simulink model "simulator_AMICAS_M2022a"  (R2024a)
settings: Solver=ode3  StartTime=0.0  StopTime=Tsim  FixedStep=ST  RelTol=1e-3
values from neighbouring files (symbols this model uses):
  alpha_G = 15.03    [anesthesia_model_AMICAS.m]
  alpha_RG = 0.33    [anesthesia_model_AMICAS.m]
  beta_M = 10.74    [anesthesia_model_AMICAS.m]
  C50N = 3.2425    [anesthesia_model_AMICAS.m]
  C50P_G = 7.66    [anesthesia_model_AMICAS.m]
  C50P_M = 7.53    [anesthesia_model_AMICAS.m]
  C50P_RG = 8.26    [anesthesia_model_AMICAS.m]
  C50Pco = 8    [hemodyn_model_AMICAS.m]
  C50Pmap = 6    [hemodyn_model_AMICAS.m]
  C50R_G = 149.62    [anesthesia_model_AMICAS.m]
  C50R_M = 160.25    [anesthesia_model_AMICAS.m]
  C50Rco = 12    [hemodyn_model_AMICAS.m]
  C50Rmap = 17    [hemodyn_model_AMICAS.m]
  Cobasis = 5    [hemodyn_model_AMICAS.m]
  E0_G = 93.97    [anesthesia_model_AMICAS.m]
  E0_M = 93.97    [anesthesia_model_AMICAS.m]
  E0_RG = 93.97    [anesthesia_model_AMICAS.m]
  Emax_G = E0_G    (= 93.97)    [anesthesia_model_AMICAS.m]
  Emax_M = E0_M    (= 93.97)    [anesthesia_model_AMICAS.m]
  Emax_RG = E0_RG    (= 93.97)    [anesthesia_model_AMICAS.m]
  EmaxPco = 5    [hemodyn_model_AMICAS.m]
  EmaxPmap = 5    [hemodyn_model_AMICAS.m]
  EmaxRco = 5    [hemodyn_model_AMICAS.m]
  EmaxRmap = 70    [hemodyn_model_AMICAS.m]
  gainPco = 10    [hemodyn_model_AMICAS.m]
  gainPmap = 15    [hemodyn_model_AMICAS.m]
  gainRco = 10    [hemodyn_model_AMICAS.m]
  gainRmap = 10    [hemodyn_model_AMICAS.m]
  gamma_G = 4.07    [anesthesia_model_AMICAS.m]
  gamma_M = 4.13    [anesthesia_model_AMICAS.m]
  gamma_RG = 3.59    [anesthesia_model_AMICAS.m]
  gammaN = 2.6677    [anesthesia_model_AMICAS.m]
  gammaPco = 4.5    [hemodyn_model_AMICAS.m]
  gammaPmap = 4.5    [hemodyn_model_AMICAS.m]
  gammaRco = 4.5    [hemodyn_model_AMICAS.m]
  gammaRmap = 4.5    [hemodyn_model_AMICAS.m]
  k0Pco = 0.81    [hemodyn_model_AMICAS.m]
  k0Pmap = 0.81    [hemodyn_model_AMICAS.m]
  k0Rco = 0.51    [hemodyn_model_AMICAS.m]
  k0Rmap = 0.31    [hemodyn_model_AMICAS.m]
  k1Pco = 0.81    [hemodyn_model_AMICAS.m]
  k1Pmap = 0.61    [hemodyn_model_AMICAS.m]
  k1Rco = 0.51    [hemodyn_model_AMICAS.m]
  k1Rmap = 0.31    [hemodyn_model_AMICAS.m]
  MAPbasis = 80    [hemodyn_model_AMICAS.m]
undefined symbols (not defined in the file or in its folder): Anest_loop, Dist_type, patient, RSM_type, Ts
libraries: cstblocks x12
settings Model: Creator=Merigo  LastModifiedBy=jarverha
settings SolverCC: AlgebraicLoopSolver=TrustRegion
settings DataIOCC: LimitDataPoints=on  SaveFormat=Array  SignalLoggingSaveFormat=ModelDataLogs  ReturnWorkspaceOutputs=off
settings OptimizationCC: BlockReduction=off  BooleanDataType=off  ReuseModelBlockBuffer=off  ExpressionDepthLimit=2147483647  LifeSpan=inf
settings DebuggingCC: SaveWithParameterizedLinksMsg=none  UnderspecifiedInitializationDetection=Classic  MergeDetectMultiDrivingBlocksExec=none  SignalResolutionControl=TryResolveAllWithWarning  MultiTaskDSMMsg=warning  MultiTaskCondExecSysMsg=none  UnconnectedInputMsg=warning  UnconnectedOutputMsg=warning  UnconnectedLineMsg=warning  StateNameClashWarn=warning  SFUnexpectedBacktrackingDiag=warning  SFNoUnconditionalDefaultTransitionDiag=warning  SFExecutionAtInitializationDiag=none  ArithmeticOperatorsInVariantConditions=warning
settings HardwareCC: ProdBitPerPointer=32  ProdBitPerSizeT=32  ProdBitPerPtrDiffT=32  ProdLargestAtomicFloat=None  ProdIntDivRoundTo=Undefined  ProdEndianess=Unspecified  ProdWordSize=32  ProdHWDeviceType=32-bit Generic  TargetUnknown=on
settings ModelReferenceCC: EnableRefExpFcnMdlSchedulingChecks=on  PropagateSignalLabelsOutOfModel=off
settings SFSimCC: SimUseLocalCustomCode=off  CustomCodeUndefinedFunction=UseInterfaceOnly
settings RTWCC: RTWUseLocalCustomCode=off  GPUComputeCapability=3.5  DLArmComputeVersion=19.05
settings CodeAppCC: StateflowObjectComments=on
settings GRTTargetCC: TargetLangStandard=C89/C90 (ANSI)
settings ConfigComp: CovMetricSettings=dw  CovSaveCumulativeToWorkspaceVar=on  CovSaveSingleToWorkspaceVar=on  CovExternalEMLEnable=off

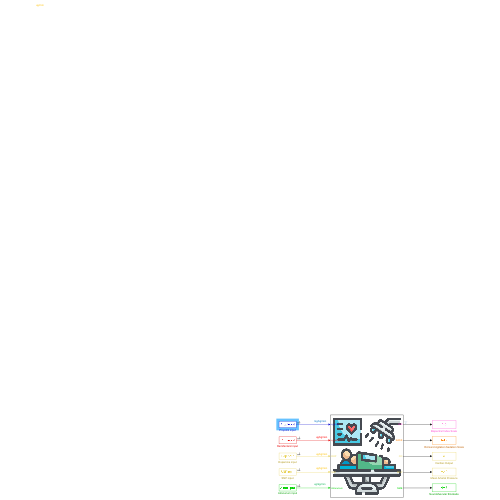
[thumbnail: Simulink's stored preview of the top-level diagram]
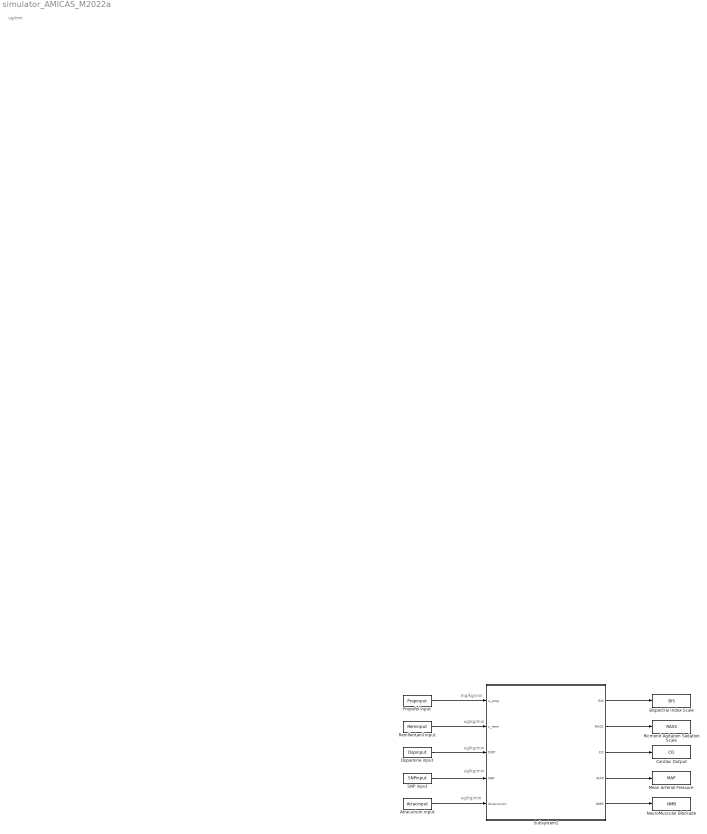
== system simulator_AMICAS_M2022a ==
  note: ug/kg/min
  note: mg/kg/min
  note: ug/min
  note: ug/kg/min
  note: ug/kg/min
  note: ug/kg/min
  Atracurium input : FromWorkspace  VariableName=Atracinput  Interpolate=off  OutputAfterFinalValue=Setting to zero
  Bispectral Index Scale : ToWorkspace  VariableName=BIS  SaveFormat=Timeseries  SampleTime=-1
  Cardiac Output : ToWorkspace  VariableName=CO  SaveFormat=Timeseries  SampleTime=-1
  Dopamine input : FromWorkspace  VariableName=Dopinput  Interpolate=off  OutputAfterFinalValue=Setting to zero
  Mean Arterial Pressure : ToWorkspace  VariableName=MAP  SaveFormat=Timeseries  SampleTime=-1
  NeuroMuscular Blockade : ToWorkspace  VariableName=NMB  SaveFormat=Timeseries  SampleTime=-1
  Propofol input : FromWorkspace  VariableName=Propinput  Interpolate=off  OutputAfterFinalValue=Setting to zero
  Remifentanil input : FromWorkspace  VariableName=Reminput  Interpolate=off  OutputAfterFinalValue=Setting to zero
  Ricmond Agitation Sedation Scale : ToWorkspace  VariableName=RASS  SaveFormat=Timeseries  SampleTime=-1
  SNP input : FromWorkspace  VariableName=SNPinput  Interpolate=off  OutputAfterFinalValue=Setting to zero
  Subsystem2 : Subsystem
      mask Display: image('$imagefile');
  wires:
  Propofol input/1 -> Subsystem2/1(u_prop)
  Subsystem2/2(RASS) -> Ricmond Agitation Sedation Scale/1
  Subsystem2/3(CO) -> Cardiac Output/1
  Subsystem2/4(MAP) -> Mean Arterial Pressure/1
  Subsystem2/5(NMB) -> NeuroMuscular Blockade/1
  Atracurium input/1 -> Subsystem2/5(Atracurium)
  Subsystem2/1(BIS) -> Bispectral Index Scale/1
  Remifentanil input/1 -> Subsystem2/2(u_remi)
  Dopamine input/1 -> Subsystem2/3(DOP)
  SNP input/1 -> Subsystem2/4(SNP)

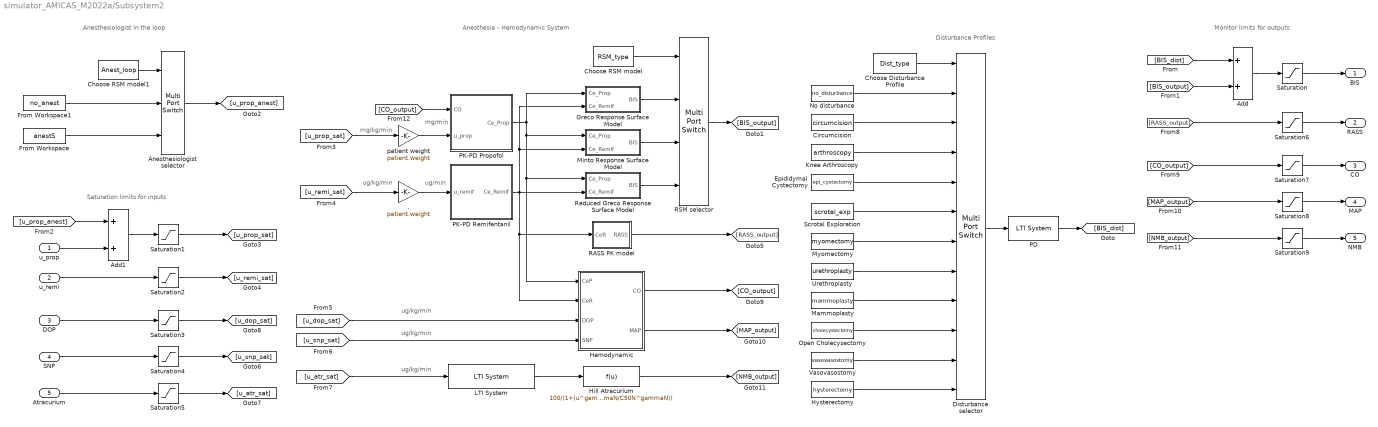
== system simulator_AMICAS_M2022a/Subsystem2 ==
  note: Disturbance Profiles
  note: Anesthesia - Hemodynamic System
  note: ug/kg/min
  note: ug/kg/min
  note: ug/kg/min
  note: ug/kg/min
  note: mg/kg/min
  note: Anesthesiologist in the loop
  note: ug/min
  note: mg/min
  note: Saturation limits for inputs
  note: Monitor limits for outputs
  u_prop : Inport
  u_remi : Inport  Port=2
  DOP : Inport  Port=3
  SNP : Inport  Port=4
  Atracurium : Inport  Port=5
  . : Gain  Gain=patient.weight
  Add : Sum
  Add1 : Sum
  Anesthesiologist selector : MultiPortSwitch  DataPortOrder=Specify indices  Inputs=2  DataPortIndices={1,2}  SaturateOnIntegerOverflow=off  InputSameDT=off
  Choose Disturbance Profile : Constant  Value=Dist_type
  Choose RSM model : Constant  Value=RSM_type
  Choose RSM model1 : Constant  Value=Anest_loop
  Circumcision : FromWorkspace  VariableName=circumcision  Interpolate=off  OutputAfterFinalValue=Setting to zero
  Disturbance selector : MultiPortSwitch  DataPortOrder=Specify indices  Inputs=10  DataPortIndices={1,2,3,4,5,6,7,8,9,10,11}  SaturateOnIntegerOverflow=off  InputSameDT=off
  Epididymal Cystectomy : FromWorkspace  VariableName=epi_cystectomy  Interpolate=off  OutputAfterFinalValue=Setting to zero
  From Workspace : FromWorkspace  VariableName=anestS
  From Workspace1 : FromWorkspace  VariableName=no_anest
  Greco Response Surface Model : Subsystem
  Hemodynamic : Subsystem
  Hill Atracurium : Fcn  Expr=100/(1+(u^gammaN/C50N^gammaN))
  Hysterectomy : FromWorkspace  VariableName=hysterectomy  Interpolate=off  OutputAfterFinalValue=Setting to zero
  Knee Arthroscopy : FromWorkspace  VariableName=arthroscopy  Interpolate=off  OutputAfterFinalValue=Setting to zero
  LTI System : cstblocks/LTI System  sys=sysNMB  IC=[]  PadeOrder=0
  Mammoplasty : FromWorkspace  VariableName=mammoplasty  Interpolate=off  OutputAfterFinalValue=Setting to zero
  Minto Response Surface Model : Subsystem
  Myomectomy : FromWorkspace  VariableName=myomectomy  Interpolate=off  OutputAfterFinalValue=Setting to zero
  No disturbance : FromWorkspace  VariableName=no_disturbance  Interpolate=off  OutputAfterFinalValue=Setting to zero
  Open Cholecysectomy : FromWorkspace  VariableName=cholecystectomy  Interpolate=off  OutputAfterFinalValue=Setting to zero
  PD : cstblocks/LTI System  sys=CPmodelP  IC=[]  PadeOrder=0
  PK-PD Propofol : Subsystem
  PK-PD Remifentanil : Subsystem
  RASS PK model : Subsystem
  RSM selector : MultiPortSwitch  DataPortOrder=Specify indices  SaturateOnIntegerOverflow=off  InputSameDT=off
  Reduced Greco Response Surface Model : Subsystem
  Saturation : Saturate  UpperLimit=100  LowerLimit=0
  Saturation1 : Saturate  UpperLimit=2.5  LowerLimit=0
  Saturation2 : Saturate  UpperLimit=4  LowerLimit=0
  Saturation3 : Saturate  UpperLimit=20  LowerLimit=0
  Saturation4 : Saturate  UpperLimit=10  LowerLimit=0
  Saturation5 : Saturate  UpperLimit=29.5  LowerLimit=0
  Saturation6 : Saturate  UpperLimit=4  LowerLimit=-5
  Saturation7 : Saturate  UpperLimit=40  LowerLimit=0
  Saturation8 : Saturate  UpperLimit=150  LowerLimit=0
  Saturation9 : Saturate  UpperLimit=100  LowerLimit=0
  Scrotal Exploration : FromWorkspace  VariableName=scrotal_exp  Interpolate=off  OutputAfterFinalValue=Setting to zero
  Urethroplasty : FromWorkspace  VariableName=urethroplasty  Interpolate=off  OutputAfterFinalValue=Setting to zero
  Vasovasostomy : FromWorkspace  VariableName=vasovasostomy  Interpolate=off  OutputAfterFinalValue=Setting to zero
  patient weight : Gain  Gain=patient.weight
  BIS : Outport
  RASS : Outport  Port=2
  CO : Outport  Port=3
  MAP : Outport  Port=4
  NMB : Outport  Port=5
  wires:
  PK-PD Remifentanil/1(Ce_Remif) -> Minto Response Surface Model/2(Ce_Remif), Greco Response Surface Model/2(Ce_Remif), Hemodynamic/2(CeR), RASS PK model/1(CeR), Reduced Greco Response Surface Model/2(Ce_Remif)
  PK-PD Propofol/1(Ce_Prop) -> Hemodynamic/1(CeP), Reduced Greco Response Surface Model/1(Ce_Prop), Minto Response Surface Model/1(Ce_Prop), Greco Response Surface Model/1(Ce_Prop)
  RASS PK model/1(RASS) -> [RASS_output]
  Hill Atracurium/1 -> [NMB_output]
  [u_atr_sat] -> LTI System/1
  LTI System/1 -> Hill Atracurium/1
  [u_dop_sat] -> Hemodynamic/3(DOP)
  [u_snp_sat] -> Hemodynamic/4(SNP)
  Hemodynamic/1(CO) -> [CO_output]
  Hemodynamic/2(MAP) -> [MAP_output]
  From Workspace/1 -> Anesthesiologist selector/3
  [u_remi_sat] -> ./1
  Reduced Greco Response Surface Model/1(BIS) -> RSM selector/4
  Greco Response Surface Model/1(BIS) -> RSM selector/2
  Minto Response Surface Model/1(BIS) -> RSM selector/3
  RSM selector/1 -> [BIS_output]
  Choose RSM model/1 -> RSM selector/1
  Add/1 -> Saturation/1
  Disturbance selector/1 -> PD/1
  No disturbance/1 -> Disturbance selector/2
  [BIS_dist] -> Add/1
  Circumcision/1 -> Disturbance selector/3
  Choose Disturbance Profile/1 -> Disturbance selector/1
  PD/1 -> [BIS_dist]
  [BIS_output] -> Add/2
  Choose RSM model1/1 -> Anesthesiologist selector/1
  Anesthesiologist selector/1 -> [u_prop_anest]
  Myomectomy/1 -> Disturbance selector/7
  Urethroplasty/1 -> Disturbance selector/8
  Mammoplasty/1 -> Disturbance selector/9
  Open Cholecysectomy/1 -> Disturbance selector/10
  From Workspace1/1 -> Anesthesiologist selector/2
  Knee Arthroscopy/1 -> Disturbance selector/4
  Hysterectomy/1 -> Disturbance selector/12
  Vasovasostomy/1 -> Disturbance selector/11
  Epididymal Cystectomy/1 -> Disturbance selector/5
  Scrotal Exploration/1 -> Disturbance selector/6
  [u_prop_sat] -> patient weight/1
  ./1 -> PK-PD Remifentanil/1(u_remif)
  patient weight/1 -> PK-PD Propofol/2(u_prop)
  Saturation/1 -> BIS/1
  u_prop/1 -> Add1/2
  Saturation1/1 -> [u_prop_sat]
  Add1/1 -> Saturation1/1
  [u_prop_anest] -> Add1/1
  u_remi/1 -> Saturation2/1
  Saturation2/1 -> [u_remi_sat]
  Saturation3/1 -> [u_dop_sat]
  DOP/1 -> Saturation3/1
  SNP/1 -> Saturation4/1
  Saturation4/1 -> [u_snp_sat]
  Atracurium/1 -> Saturation5/1
  Saturation5/1 -> [u_atr_sat]
  [RASS_output] -> Saturation6/1
  Saturation6/1 -> RASS/1
  Saturation7/1 -> CO/1
  [CO_output] -> Saturation7/1
  Saturation8/1 -> MAP/1
  [MAP_output] -> Saturation8/1
  Saturation9/1 -> NMB/1
  [NMB_output] -> Saturation9/1
  [CO_output] -> PK-PD Propofol/1(CO)

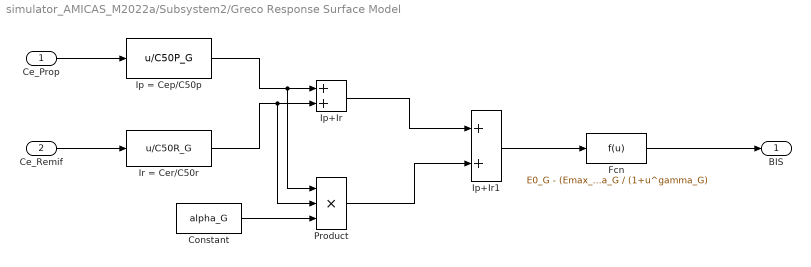
== system simulator_AMICAS_M2022a/Subsystem2/Greco Response Surface Model ==
  Ce_Prop : Inport
  Ce_Remif : Inport  Port=2
  Constant : Constant  Value=alpha_G
  Fcn : Fcn  Expr=E0_G - (Emax_G) * u^gamma_G / (1+u^gamma_G)
  Ip = Cep/C50p : Fcn  Expr=u/C50P_G
  Ip+Ir : Sum
  Ip+Ir1 : Sum
  Ir = Cer/C50r : Fcn  Expr=u/C50R_G
  Product : Product  Inputs=3
  BIS : Outport
  wires:
  Fcn/1 -> BIS/1
  Ip+Ir1/1 -> Fcn/1
  Ir = Cer/C50r/1 -> Product/2, Ip+Ir/2
  Ip = Cep/C50p/1 -> Product/1, Ip+Ir/1
  Ce_Remif/1 -> Ir = Cer/C50r/1
  Ce_Prop/1 -> Ip = Cep/C50p/1
  Ip+Ir/1 -> Ip+Ir1/1
  Constant/1 -> Product/3
  Product/1 -> Ip+Ir1/2

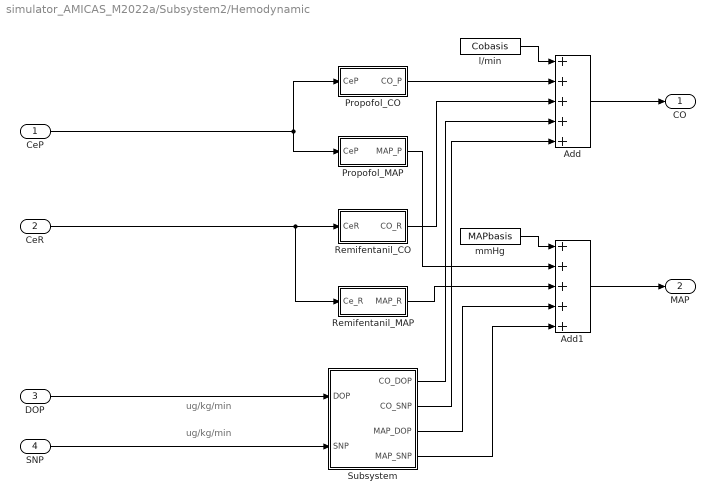
== system simulator_AMICAS_M2022a/Subsystem2/Hemodynamic ==
  note: ug/kg/min
  note: ug/kg/min
  CeP : Inport
  CeR : Inport  Port=2
  DOP : Inport  Port=3
  SNP : Inport  Port=4
  Add : Sum  Inputs=+++++
  Add1 : Sum  Inputs=+++++
  Propofol_CO : Subsystem
  Propofol_MAP : Subsystem
  Remifentanil_CO : Subsystem
  Remifentanil_MAP : Subsystem
  Subsystem : Subsystem
  l/min : Constant  Value=Cobasis  SampleTime=Ts
  mmHg : Constant  Value=MAPbasis  SampleTime=Ts
  CO : Outport
  MAP : Outport  Port=2
  wires:
  DOP/1 -> Subsystem/1(DOP)
  SNP/1 -> Subsystem/2(SNP)
  Subsystem/1(CO_DOP) -> Add/4
  Propofol_CO/1(CO_P) -> Add/2
  Subsystem/3(MAP_DOP) -> Add1/4
  CeP/1 -> Propofol_CO/1(CeP), Propofol_MAP/1(CeP)
  Subsystem/2(CO_SNP) -> Add/5
  CeR/1 -> Remifentanil_MAP/1(Ce_R), Remifentanil_CO/1(CeR)
  Propofol_MAP/1(MAP_P) -> Add1/2
  Remifentanil_CO/1(CO_R) -> Add/3
  Add/1 -> CO/1
  Add1/1 -> MAP/1
  mmHg/1 -> Add1/1
  Subsystem/4(MAP_SNP) -> Add1/5
  l/min/1 -> Add/1
  Remifentanil_MAP/1(MAP_R) -> Add1/3

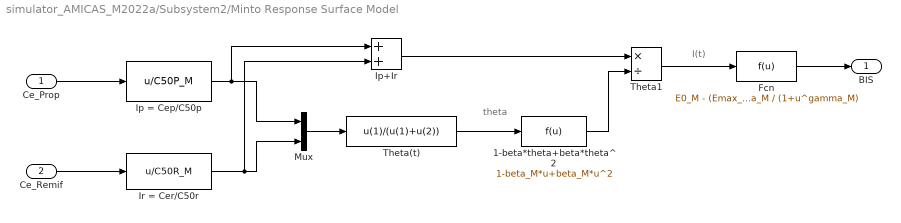
== system simulator_AMICAS_M2022a/Subsystem2/Minto Response Surface Model ==
  note: I(t)
  note: theta
  Ce_Prop : Inport
  Ce_Remif : Inport  Port=2
  1-beta*theta+beta*theta^2 : Fcn  Expr=1-beta_M*u+beta_M*u^2
  Fcn : Fcn  Expr=E0_M - (Emax_M)*u^gamma_M / (1+u^gamma_M)
  Ip = Cep/C50p : Fcn  Expr=u/C50P_M
  Ip+Ir : Sum
  Ir = Cer/C50r : Fcn  Expr=u/C50R_M
  Mux : Mux  Inputs=2
  Theta(t) : Fcn  Expr=u(1)/(u(1)+u(2))
  Theta1 : Product  Inputs=*/
  BIS : Outport
  wires:
  Ce_Prop/1 -> Ip = Cep/C50p/1
  Ce_Remif/1 -> Ir = Cer/C50r/1
  Ip = Cep/C50p/1 -> Mux/1, Ip+Ir/1
  Ir = Cer/C50r/1 -> Mux/2, Ip+Ir/2
  Mux/1 -> Theta(t)/1
  Ip+Ir/1 -> Theta1/1
  Theta(t)/1 -> 1-beta*theta+beta*theta^2/1
  1-beta*theta+beta*theta^2/1 -> Theta1/2
  Theta1/1 -> Fcn/1
  Fcn/1 -> BIS/1

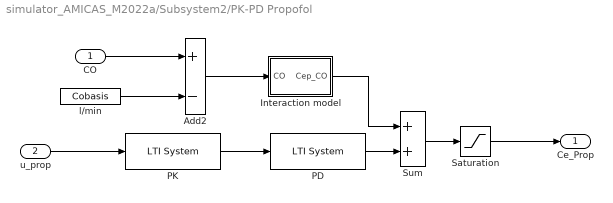
== system simulator_AMICAS_M2022a/Subsystem2/PK-PD Propofol ==
  CO : Inport
  u_prop : Inport  Port=2
  Add2 : Sum  Inputs=+-
  Interaction model : Subsystem
  PD : cstblocks/LTI System  sys=CPmodelP  IC=[]  PadeOrder=0
  PK : cstblocks/LTI System  sys=PKmodelP  IC=[]  PadeOrder=0
  Saturation : Saturate  UpperLimit=Inf  LowerLimit=0.001  ZeroCross=off
  Sum : Sum
  l/min : Constant  Value=Cobasis  SampleTime=Ts
  Ce_Prop : Outport
  wires:
  u_prop/1 -> PK/1
  PD/1 -> Sum/2
  PK/1 -> PD/1
  Saturation/1 -> Ce_Prop/1
  l/min/1 -> Add2/2
  Add2/1 -> Interaction model/1(CO)
  Sum/1 -> Saturation/1
  CO/1 -> Add2/1
  Interaction model/1(Cep_CO) -> Sum/1

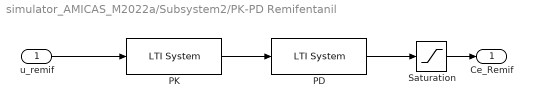
== system simulator_AMICAS_M2022a/Subsystem2/PK-PD Remifentanil ==
  u_remif : Inport
  PD : cstblocks/LTI System  sys=CPmodelR  IC=[]  PadeOrder=0
  PK : cstblocks/LTI System  sys=PKmodelR  IC=[]  PadeOrder=0
  Saturation : Saturate  UpperLimit=Inf  LowerLimit=0.001  ZeroCross=off
  Ce_Remif : Outport
  wires:
  PK/1 -> PD/1
  u_remif/1 -> PK/1
  PD/1 -> Saturation/1
  Saturation/1 -> Ce_Remif/1

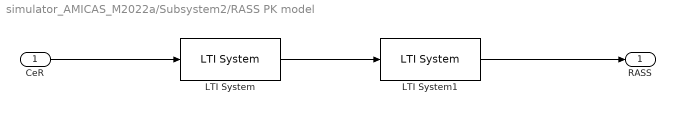
== system simulator_AMICAS_M2022a/Subsystem2/RASS PK model ==
  CeR : Inport
  LTI System : cstblocks/LTI System  sys=sysRASS1  IC=[]  PadeOrder=0
  LTI System1 : cstblocks/LTI System  sys=sysRASS2  IC=[]  PadeOrder=0
  RASS : Outport
  wires:
  CeR/1 -> LTI System/1
  LTI System/1 -> LTI System1/1
  LTI System1/1 -> RASS/1

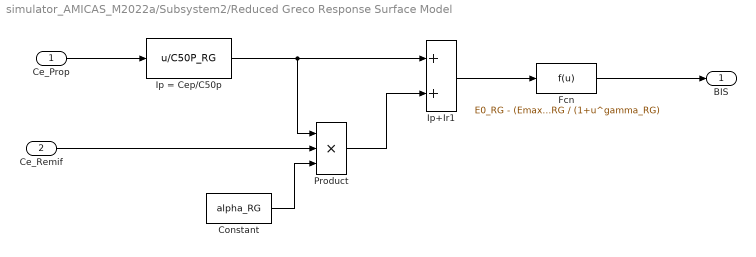
== system simulator_AMICAS_M2022a/Subsystem2/Reduced Greco Response Surface Model ==
  Ce_Prop : Inport
  Ce_Remif : Inport  Port=2
  Constant : Constant  Value=alpha_RG
  Fcn : Fcn  Expr=E0_RG - (Emax_RG ) * u^gamma_RG / (1+u^gamma_RG)
  Ip = Cep/C50p : Fcn  Expr=u/C50P_RG
  Ip+Ir1 : Sum
  Product : Product  Inputs=3
  BIS : Outport
  wires:
  Fcn/1 -> BIS/1
  Ip+Ir1/1 -> Fcn/1
  Ce_Remif/1 -> Product/2
  Ce_Prop/1 -> Ip = Cep/C50p/1
  Ip = Cep/C50p/1 -> Product/1, Ip+Ir1/1
  Constant/1 -> Product/3
  Product/1 -> Ip+Ir1/2

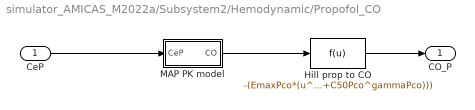
== system simulator_AMICAS_M2022a/Subsystem2/Hemodynamic/Propofol_CO ==
  CeP : Inport
  Hill prop to CO : Fcn  Expr=-(EmaxPco*(u^gammaPco/(u^gammaPco+C50Pco^gammaPco)))
  MAP PK model : Subsystem
  CO_P : Outport  VectorParamsAs1DForOutWhenUnconnected=off
  wires:
  MAP PK model/1(CO) -> Hill prop to CO/1
  CeP/1 -> MAP PK model/1(CeP)
  Hill prop to CO/1 -> CO_P/1

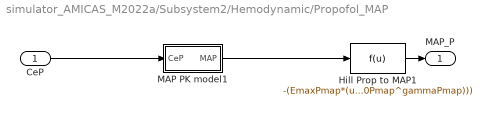
== system simulator_AMICAS_M2022a/Subsystem2/Hemodynamic/Propofol_MAP ==
  CeP : Inport
  Hill Prop to MAP1 : Fcn  Expr=-(EmaxPmap*(u^gammaPmap/(u^gammaPmap+C50Pmap^gammaPmap)))
  MAP PK model1 : Subsystem
  MAP_P : Outport  VectorParamsAs1DForOutWhenUnconnected=off
  wires:
  MAP PK model1/1(MAP) -> Hill Prop to MAP1/1
  CeP/1 -> MAP PK model1/1(CeP)
  Hill Prop to MAP1/1 -> MAP_P/1

== system simulator_AMICAS_M2022a/Subsystem2/Hemodynamic/Remifentanil_CO ==
  CeR : Inport
  Hill Remifentanil to CO : Fcn  Expr=EmaxRco*(u^gammaRco/(u^gammaRco+C50Rco^gammaRco))
  MAP PK model2 : Subsystem
  CO_R : Outport  VectorParamsAs1DForOutWhenUnconnected=off
  wires:
  CeR/1 -> MAP PK model2/1(CeR)
  MAP PK model2/1(CO) -> Hill Remifentanil to CO/1
  Hill Remifentanil to CO/1 -> CO_R/1

== system simulator_AMICAS_M2022a/Subsystem2/Hemodynamic/Remifentanil_MAP ==
  Ce_R : Inport
  Hill Remi MAP : Fcn  Expr=-(EmaxRmap*(u^gammaRmap/(u^gammaRmap+C50Rmap^gammaRmap)))
  MAP PK model3 : Subsystem
  MAP_R : Outport  VectorParamsAs1DForOutWhenUnconnected=off
  wires:
  Ce_R/1 -> MAP PK model3/1(CeR)
  MAP PK model3/1(MAP) -> Hill Remi MAP/1
  Hill Remi MAP/1 -> MAP_R/1

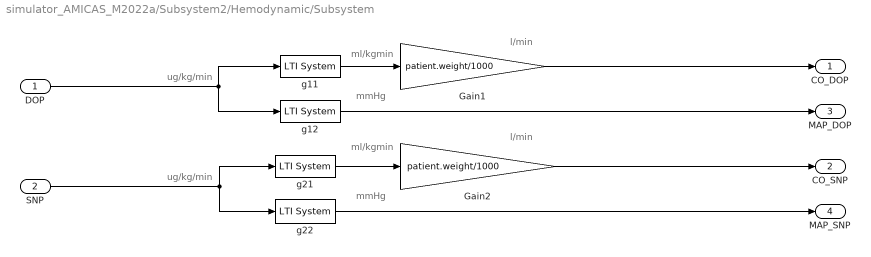
== system simulator_AMICAS_M2022a/Subsystem2/Hemodynamic/Subsystem ==
  note: ml/kgmin
  note: l/min
  note: ug/kg/min
  note: mmHg
  note: mmHg
  note: ug/kg/min
  note: ml/kgmin
  note: l/min
  DOP : Inport
  SNP : Inport  Port=2
  Gain1 : Gain  Gain=patient.weight/1000
  Gain2 : Gain  Gain=patient.weight/1000
  g11 : cstblocks/LTI System  sys=g11  IC=[]  PadeOrder=0
  g12 : cstblocks/LTI System  sys=g12  IC=[]  PadeOrder=0
  g21 : cstblocks/LTI System  sys=g21  IC=[]  PadeOrder=0
  g22 : cstblocks/LTI System  sys=g22  IC=[]  PadeOrder=0
  CO_DOP : Outport
  CO_SNP : Outport  Port=2
  MAP_DOP : Outport  Port=3
  MAP_SNP : Outport  Port=4
  wires:
  Gain1/1 -> CO_DOP/1
  SNP/1 -> g22/1, g21/1
  g12/1 -> MAP_DOP/1
  g22/1 -> MAP_SNP/1
  g21/1 -> Gain2/1
  DOP/1 -> g12/1, g11/1
  g11/1 -> Gain1/1
  Gain2/1 -> CO_SNP/1

== system simulator_AMICAS_M2022a/Subsystem2/PK-PD Propofol/Interaction model ==
  CO : Inport
  Transfer Fcn : TransferFcn  Numerator=[-0.35]  Denominator=[300 1]
  Cep_CO : Outport
  wires:
  CO/1 -> Transfer Fcn/1
  Transfer Fcn/1 -> Cep_CO/1

== system simulator_AMICAS_M2022a/Subsystem2/Hemodynamic/Propofol_CO/MAP PK model ==
  CeP : Inport
  Transfer Fcn : TransferFcn  Numerator=[0.7]  Denominator=[k1Pco*gainPco k0Pco]
  CO : Outport
  wires:
  Transfer Fcn/1 -> CO/1
  CeP/1 -> Transfer Fcn/1

== system simulator_AMICAS_M2022a/Subsystem2/Hemodynamic/Propofol_MAP/MAP PK model1 ==
  CeP : Inport
  Transfer Fcn : TransferFcn  Denominator=[k1Pmap*gainPmap k0Pmap]
  MAP : Outport
  wires:
  Transfer Fcn/1 -> MAP/1
  CeP/1 -> Transfer Fcn/1

== system simulator_AMICAS_M2022a/Subsystem2/Hemodynamic/Remifentanil_CO/MAP PK model2 ==
  CeR : Inport
  Transfer Fcn : TransferFcn  Denominator=[k1Rco*gainRco k0Rco]
  CO : Outport
  wires:
  Transfer Fcn/1 -> CO/1
  CeR/1 -> Transfer Fcn/1

== system simulator_AMICAS_M2022a/Subsystem2/Hemodynamic/Remifentanil_MAP/MAP PK model3 ==
  CeR : Inport
  Transfer Fcn : TransferFcn  Denominator=[k1Rmap*gainRmap k0Rmap]
  MAP : Outport
  wires:
  Transfer Fcn/1 -> MAP/1
  CeR/1 -> Transfer Fcn/1
